simulink model "VTOL_quadplane"  (R2026a)
settings: Solver=ode1  StopTime=120  FixedStep=1/60  MaxStep=0.01
undefined symbols (not defined in the file or in its folder): op_trim, params, Receive, Send
libraries: slpidlib x32, simulink_extras x11, simulink x2, aerolibfltsims x2, aerolibobsolete x1, sim3dlib x1, uavsim3dlib x1
(part 2 of 4)

== system VTOL_quadplane/Gravity_forces ==
  DCM : Inport
  Constant2 : Constant  Value=[0;0;params.geometric.mass*params.constants.g]
  MatrixMultiply : Product  Multiplication=Matrix(*)
  Gravity_forces : Outport
  wires:
  DCM/1 -> MatrixMultiply/1
  Constant2/1 -> MatrixMultiply/2
  MatrixMultiply/1 -> Gravity_forces/1

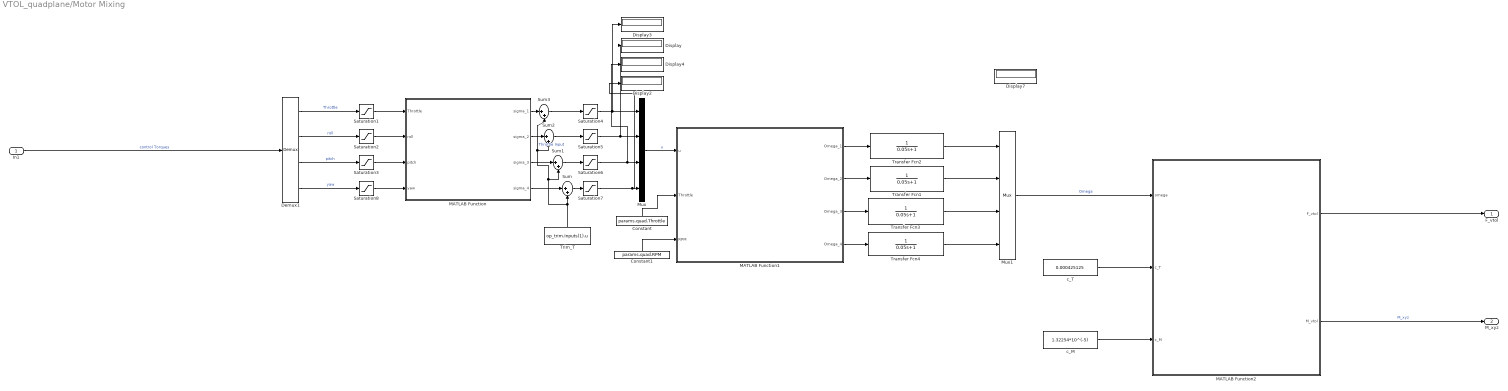
== system VTOL_quadplane/Motor Mixing ==
  In1 : Inport
  Constant : Constant  Value=params.quad.Throttle
  Constant1 : Constant  Value=params.quad.RPM
  Demux1 : Demux
  Display{,2..4,7} (5 alike) : Display
  MATLAB Function : MATLAB Function  TreatAsAtomicUnit=on
  MATLAB Function1 : MATLAB Function  TreatAsAtomicUnit=on
  MATLAB Function2 : MATLAB Function  TreatAsAtomicUnit=on
  Mux : Mux
  Mux1 : Mux
  Saturation1 : Saturate  UpperLimit=0.15  LowerLimit=-0.15
  Saturation2 : Saturate  UpperLimit=0.15  LowerLimit=-0.15
  Saturation3 : Saturate  UpperLimit=0.15  LowerLimit=-0.15
  Saturation{4..7} (4 alike) : Saturate  UpperLimit=0.9  LowerLimit=0.1
  Saturation8 : Saturate  UpperLimit=0.05  LowerLimit=-0.05
  Sum{,1..3} (4 alike) : Sum  Inputs=|++
  Transfer Fcn{1..4} (4 alike) : TransferFcn  Denominator=[0.05 1]
  Trim_T : Constant  Value=op_trim.Inputs(1).u
  c_M : Constant  Value=1.32254*10^(-5)
  c_T : Constant  Value=0.000425125
  F_vtol : Outport
  M_xyz : Outport  Port=2
  wires:
  Saturation4/1 -> Display3/1, Mux/1
  Demux1/4 -> Saturation8/1  "yaw"
  Constant/1 -> MATLAB Function1/2(Throttle)
  MATLAB Function1/3(Omega_3) -> Transfer Fcn3/1
  MATLAB Function1/1(Omega_1) -> Transfer Fcn2/1
  MATLAB Function1/2(Omega_2) -> Transfer Fcn1/1
  MATLAB Function1/4(Omega_4) -> Transfer Fcn4/1
  Mux1/1 -> MATLAB Function2/1(omega)  "Omega"
  Saturation7/1 -> Display2/1, Mux/4
  Demux1/1 -> Saturation1/1  "Throttle"
  Demux1/3 -> Saturation3/1  "pitch"
  MATLAB Function2/2(M_vtol) -> M_xyz/1  "M_xyz"
  Mux/1 -> MATLAB Function1/1(u)  "u"
  Demux1/2 -> Saturation2/1  "roll"
  In1/1 -> Demux1/1  "control Torques"
  Saturation5/1 -> Display/1, Mux/2
  Constant1/1 -> MATLAB Function1/3(RPM)
  Saturation6/1 -> Display4/1, Mux/3
  c_M/1 -> MATLAB Function2/3(c_M)
  c_T/1 -> MATLAB Function2/2(c_T)
  MATLAB Function2/1(F_vtol) -> F_vtol/1
  Transfer Fcn2/1 -> Mux1/1
  Transfer Fcn1/1 -> Mux1/2
  Transfer Fcn3/1 -> Mux1/3
  Transfer Fcn4/1 -> Mux1/4
  Sum/1 -> Saturation7/1
  Trim_T/1 -> Sum1/2, Sum3/2, Sum2/2, Sum/2  "Throttle Input"
  MATLAB Function/1(sigma_1) -> Sum3/1
  MATLAB Function/2(sigma_2) -> Sum2/1
  MATLAB Function/3(sigma_3) -> Sum1/1
  MATLAB Function/4(sigma_4) -> Sum/1
  Sum1/1 -> Saturation6/1
  Sum2/1 -> Saturation5/1
  Sum3/1 -> Saturation4/1
  Saturation1/1 -> MATLAB Function/1(Throttle)
  Saturation2/1 -> MATLAB Function/2(roll)
  Saturation3/1 -> MATLAB Function/3(pitch)
  Saturation8/1 -> MATLAB Function/4(yaw)

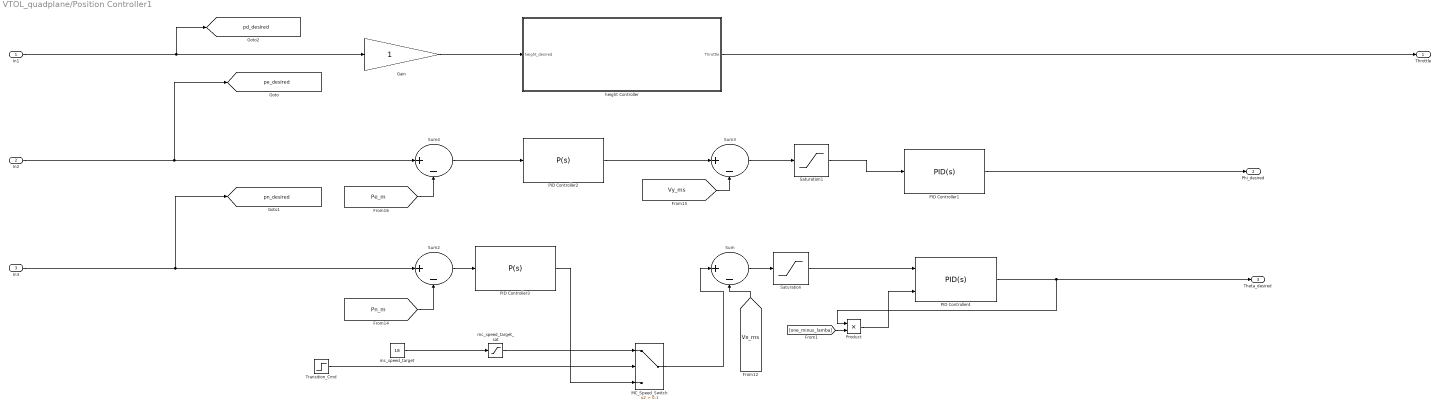
== system VTOL_quadplane/Position Controller1 ==
  In1 : Inport
  In2 : Inport  Port=2
  In3 : Inport  Port=3
  Gain : Gain
  MC_Speed_Switch : Switch  Criteria=u2 > Threshold  Threshold=0.1  SaturateOnIntegerOverflow=off  InputSameDT=off
  PID Controller1 : slpidlib/PID Controller  Controller=PID  Form=Parallel  TimeDomain=Continuous-time  UseExternalTs=off  SampleTime=-1  IntegratorMethod=Forward Euler  FilterMethod=Forward Euler  ControllerParametersSource=internal  P=0.103  I=0.0188  UseKiTs=off  D=0.0191  UseExternalDerivativeSource=off  N=100  UseFilter=on  TunerSelectOption=Transfer Function Based (PID Tuner App)  InitialConditionSource=internal  InitialConditionForIntegrator=0  InitialConditionForFilter=0  DifferentiatorICPrevScaledInput=0  ExternalReset=none  TrackingMode=off  Kt=1  LimitOutput=on  SatLimitsSource=internal  UpperSaturationLimit=deg2rad(25)  LowerSaturationLimit=-deg2rad(25)  LinearizeAsGain=on  AntiWindupMode=back-calculation  Kb=1  LimitIntegrator=off  UpperIntegratorSaturationLimit=inf  LowerIntegratorSaturationLimit=-inf  POutMin=[]  POutMax=[]  IOutMin=[]  IOutMax=[]  DOutMin=[]  DOutMax=[]  NOutMin=[]  NOutMax=[]  SumOutMin=[]  SumOutMax=[]  SaturationOutMin=[]  SaturationOutMax=[]  PParamMin=[]  PParamMax=[]  IParamMin=[]  IParamMax=[]  DParamMin=[]  DParamMax=[]  NParamMin=[]  NParamMax=[]  KbParamMin=[]  KbParamMax=[]  KtParamMin=[]  KtParamMax=[]  KbOutMin=[]  KbOutMax=[]  KtOutMin=[]  KtOutMax=[]  IntegratorOutMin=[]  IntegratorOutMax=[]  FilterOutMin=[]  FilterOutMax=[]  SumI1OutMin=[]  SumI1OutMax=[]  SumI2OutMin=[]  SumI2OutMax=[]  SumI3OutMin=[]  SumI3OutMax=[]  SumI4OutMin=[]  SumI4OutMax=[]  SumDOutMin=[]  SumDOutMax=[]  DifferentiatorOutMin=[]  DifferentiatorOutMax=[]  FilterDiffOutCoefMin=[]  FilterDiffOutCoefMax=[]  ReciprocalOutMin=[]  ReciprocalOutMax=[]  SumDenOutMin=[]  SumDenOutMax=[]  SumNumOutMin=[]  SumNumOutMax=[]  DivideOutMin=[]  DivideOutMax=[]  UdiffTsProdOutMin=[]  UdiffTsProdOutMax=[]  NTsProdOutMin=[]  NTsProdOutMax=[]  UintegralTsProdOutMin=[]  UintegralTsProdOutMax=[]  UngainTsProdOutMin=[]  UngainTsProdOutMax=[]  ClampingZeroOutDataTypeStr=Inherit: Inherit via back propagation  ClampingZeroOutMin=[]  ClampingZeroOutMax=[]  FilterDenConstantOutDataTypeStr=Inherit: Inherit via back propagation  FilterDenConstantOutMin=[]  FilterDenConstantOutMax=[]  PCopyOutDataTypeStr=Inherit: Inherit via back propagation  PCopyOutMin=[]  PCopyOutMax=[]  NCopyOutDataTypeStr=Inherit: Inherit via back propagation  NCopyOutMin=[]  NCopyOutMax=[]  IntegratorContinuousStateAttributes=''  IntegratorStateMustResolveToSignalObject=off  IntegratorRTWStateStorageClass=Auto  FilterContinuousStateAttributes=''  FilterStateMustResolveToSignalObject=off  FilterRTWStateStorageClass=Auto  ParallelPVariant=InternalParameters  IdealPVariant=Disabled  IVariant=InternalParameters  DVariant=InternalParameters  IntegratorVariant=Continuous  SatVariant=Enabled  AWVariant=BackCalculation  PCopyVariant=Disabled  TRVariant=Disabled  FdbkBlocksVariant=Forward  IdealPFdbkVariant=Disabled  SatFdbkVariant=Disabled  DerivativeFilterVariant=ContFilter  NVariant=InternalParameters  NCopyVariant=Disabled  FilterICVariant=InternalICsFilter  IntegratorICVariant=InternalICs  ExternalResetVariant=Disabled  TRSumVariant=Passthrough  SumFdbkVariant=Disabled  SumVariant=Sum_PID  TsampFilterVariant=InternalTs  TsampNgainVariant=Passthrough  TsampIntegralVariant=Disabled_SignalSpec  ExternalSaturationOutDataTypeStr=Inherit: Same as second input  DerivativeSourceVariant=ErrorSignal  PreIntVariant=InternalPreInt
  PID Controller2 : slpidlib/PID Controller  Controller=P  Form=Parallel  TimeDomain=Continuous-time  UseExternalTs=off  SampleTime=-1  IntegratorMethod=Forward Euler  FilterMethod=Forward Euler  ControllerParametersSource=internal  P=0.266  I=1  UseKiTs=off  D=0.212  UseExternalDerivativeSource=off  N=100  UseFilter=on  TunerSelectOption=Transfer Function Based (PID Tuner App)  InitialConditionSource=internal  InitialConditionForIntegrator=0  InitialConditionForFilter=0  DifferentiatorICPrevScaledInput=0  ExternalReset=none  TrackingMode=off  Kt=1  LimitOutput=off  SatLimitsSource=internal  UpperSaturationLimit=inf  LowerSaturationLimit=-inf  LinearizeAsGain=on  AntiWindupMode=none  Kb=1  LimitIntegrator=off  UpperIntegratorSaturationLimit=inf  LowerIntegratorSaturationLimit=-inf  POutMin=[]  POutMax=[]  IOutMin=[]  IOutMax=[]  DOutMin=[]  DOutMax=[]  NOutMin=[]  NOutMax=[]  SumOutMin=[]  SumOutMax=[]  SaturationOutMin=[]  SaturationOutMax=[]  PParamMin=[]  PParamMax=[]  IParamMin=[]  IParamMax=[]  DParamMin=[]  DParamMax=[]  NParamMin=[]  NParamMax=[]  KbParamMin=[]  KbParamMax=[]  KtParamMin=[]  KtParamMax=[]  KbOutMin=[]  KbOutMax=[]  KtOutMin=[]  KtOutMax=[]  IntegratorOutMin=[]  IntegratorOutMax=[]  FilterOutMin=[]  FilterOutMax=[]  SumI1OutMin=[]  SumI1OutMax=[]  SumI2OutMin=[]  SumI2OutMax=[]  SumI3OutMin=[]  SumI3OutMax=[]  SumI4OutMin=[]  SumI4OutMax=[]  SumDOutMin=[]  SumDOutMax=[]  DifferentiatorOutMin=[]  DifferentiatorOutMax=[]  FilterDiffOutCoefMin=[]  FilterDiffOutCoefMax=[]  ReciprocalOutMin=[]  ReciprocalOutMax=[]  SumDenOutMin=[]  SumDenOutMax=[]  SumNumOutMin=[]  SumNumOutMax=[]  DivideOutMin=[]  DivideOutMax=[]  UdiffTsProdOutMin=[]  UdiffTsProdOutMax=[]  NTsProdOutMin=[]  NTsProdOutMax=[]  UintegralTsProdOutMin=[]  UintegralTsProdOutMax=[]  UngainTsProdOutMin=[]  UngainTsProdOutMax=[]  ClampingZeroOutDataTypeStr=Inherit: Inherit via back propagation  ClampingZeroOutMin=[]  ClampingZeroOutMax=[]  FilterDenConstantOutDataTypeStr=Inherit: Inherit via back propagation  FilterDenConstantOutMin=[]  FilterDenConstantOutMax=[]  PCopyOutDataTypeStr=Inherit: Inherit via back propagation  PCopyOutMin=[]  PCopyOutMax=[]  NCopyOutDataTypeStr=Inherit: Inherit via back propagation  NCopyOutMin=[]  NCopyOutMax=[]  IntegratorContinuousStateAttributes=''  IntegratorStateMustResolveToSignalObject=off  IntegratorRTWStateStorageClass=Auto  FilterContinuousStateAttributes=''  FilterStateMustResolveToSignalObject=off  FilterRTWStateStorageClass=Auto  ParallelPVariant=InternalParameters  IdealPVariant=Disabled  IVariant=Disabled  DVariant=Disabled  IntegratorVariant=Disabled  SatVariant=Disabled  AWVariant=Disabled  PCopyVariant=Disabled  TRVariant=Disabled  FdbkBlocksVariant=Forward  IdealPFdbkVariant=Disabled  SatFdbkVariant=Disabled  DerivativeFilterVariant=Disabled  NVariant=Disabled  NCopyVariant=Disabled_SignalSpec  FilterICVariant=Disabled  IntegratorICVariant=Disabled  ExternalResetVariant=Disabled  TRSumVariant=Passthrough  SumFdbkVariant=Disabled  SumVariant=Passthrough_P  TsampFilterVariant=InternalTs  TsampNgainVariant=Passthrough  TsampIntegralVariant=Disabled_SignalSpec  ExternalSaturationOutDataTypeStr=Inherit: Same as second input  DerivativeSourceVariant=Disabled  PreIntVariant=InternalPreInt
  PID Controller3 : slpidlib/PID Controller  Controller=P  Form=Parallel  TimeDomain=Continuous-time  UseExternalTs=off  SampleTime=-1  IntegratorMethod=Forward Euler  FilterMethod=Forward Euler  ControllerParametersSource=internal  P=0.266  I=1  UseKiTs=off  D=0.1  UseExternalDerivativeSource=off  N=100  UseFilter=on  TunerSelectOption=Transfer Function Based (PID Tuner App)  InitialConditionSource=internal  InitialConditionForIntegrator=0  InitialConditionForFilter=0  DifferentiatorICPrevScaledInput=0  ExternalReset=none  TrackingMode=off  Kt=1  LimitOutput=off  SatLimitsSource=internal  UpperSaturationLimit=inf  LowerSaturationLimit=-inf  LinearizeAsGain=on  AntiWindupMode=none  Kb=1  LimitIntegrator=off  UpperIntegratorSaturationLimit=inf  LowerIntegratorSaturationLimit=-inf  POutMin=[]  POutMax=[]  IOutMin=[]  IOutMax=[]  DOutMin=[]  DOutMax=[]  NOutMin=[]  NOutMax=[]  SumOutMin=[]  SumOutMax=[]  SaturationOutMin=[]  SaturationOutMax=[]  PParamMin=[]  PParamMax=[]  IParamMin=[]  IParamMax=[]  DParamMin=[]  DParamMax=[]  NParamMin=[]  NParamMax=[]  KbParamMin=[]  KbParamMax=[]  KtParamMin=[]  KtParamMax=[]  KbOutMin=[]  KbOutMax=[]  KtOutMin=[]  KtOutMax=[]  IntegratorOutMin=[]  IntegratorOutMax=[]  FilterOutMin=[]  FilterOutMax=[]  SumI1OutMin=[]  SumI1OutMax=[]  SumI2OutMin=[]  SumI2OutMax=[]  SumI3OutMin=[]  SumI3OutMax=[]  SumI4OutMin=[]  SumI4OutMax=[]  SumDOutMin=[]  SumDOutMax=[]  DifferentiatorOutMin=[]  DifferentiatorOutMax=[]  FilterDiffOutCoefMin=[]  FilterDiffOutCoefMax=[]  ReciprocalOutMin=[]  ReciprocalOutMax=[]  SumDenOutMin=[]  SumDenOutMax=[]  SumNumOutMin=[]  SumNumOutMax=[]  DivideOutMin=[]  DivideOutMax=[]  UdiffTsProdOutMin=[]  UdiffTsProdOutMax=[]  NTsProdOutMin=[]  NTsProdOutMax=[]  UintegralTsProdOutMin=[]  UintegralTsProdOutMax=[]  UngainTsProdOutMin=[]  UngainTsProdOutMax=[]  ClampingZeroOutDataTypeStr=Inherit: Inherit via back propagation  ClampingZeroOutMin=[]  ClampingZeroOutMax=[]  FilterDenConstantOutDataTypeStr=Inherit: Inherit via back propagation  FilterDenConstantOutMin=[]  FilterDenConstantOutMax=[]  PCopyOutDataTypeStr=Inherit: Inherit via back propagation  PCopyOutMin=[]  PCopyOutMax=[]  NCopyOutDataTypeStr=Inherit: Inherit via back propagation  NCopyOutMin=[]  NCopyOutMax=[]  IntegratorContinuousStateAttributes=''  IntegratorStateMustResolveToSignalObject=off  IntegratorRTWStateStorageClass=Auto  FilterContinuousStateAttributes=''  FilterStateMustResolveToSignalObject=off  FilterRTWStateStorageClass=Auto  ParallelPVariant=InternalParameters  IdealPVariant=Disabled  IVariant=Disabled  DVariant=Disabled  IntegratorVariant=Disabled  SatVariant=Disabled  AWVariant=Disabled  PCopyVariant=Disabled  TRVariant=Disabled  FdbkBlocksVariant=Forward  IdealPFdbkVariant=Disabled  SatFdbkVariant=Disabled  DerivativeFilterVariant=Disabled  NVariant=Disabled  NCopyVariant=Disabled_SignalSpec  FilterICVariant=Disabled  IntegratorICVariant=Disabled  ExternalResetVariant=Disabled  TRSumVariant=Passthrough  SumFdbkVariant=Disabled  SumVariant=Passthrough_P  TsampFilterVariant=InternalTs  TsampNgainVariant=Passthrough  TsampIntegralVariant=Disabled_SignalSpec  ExternalSaturationOutDataTypeStr=Inherit: Same as second input  DerivativeSourceVariant=Disabled  PreIntVariant=InternalPreInt
  PID Controller4 : slpidlib/PID Controller  Controller=PID  Form=Parallel  TimeDomain=Continuous-time  UseExternalTs=off  SampleTime=-1  IntegratorMethod=Forward Euler  FilterMethod=Forward Euler  ControllerParametersSource=internal  P=-0.102  I=-0.0188  UseKiTs=off  D=-0.0191  UseExternalDerivativeSource=off  N=100  UseFilter=on  TunerSelectOption=Transfer Function Based (PID Tuner App)  InitialConditionSource=internal  InitialConditionForIntegrator=0  InitialConditionForFilter=0  DifferentiatorICPrevScaledInput=0  ExternalReset=none  TrackingMode=on  Kt=1  LimitOutput=on  SatLimitsSource=internal  UpperSaturationLimit=deg2rad(25)  LowerSaturationLimit=-deg2rad(25)  LinearizeAsGain=on  AntiWindupMode=back-calculation  Kb=1  LimitIntegrator=off  UpperIntegratorSaturationLimit=inf  LowerIntegratorSaturationLimit=-inf  POutMin=[]  POutMax=[]  IOutMin=[]  IOutMax=[]  DOutMin=[]  DOutMax=[]  NOutMin=[]  NOutMax=[]  SumOutMin=[]  SumOutMax=[]  SaturationOutMin=[]  SaturationOutMax=[]  PParamMin=[]  PParamMax=[]  IParamMin=[]  IParamMax=[]  DParamMin=[]  DParamMax=[]  NParamMin=[]  NParamMax=[]  KbParamMin=[]  KbParamMax=[]  KtParamMin=[]  KtParamMax=[]  KbOutMin=[]  KbOutMax=[]  KtOutMin=[]  KtOutMax=[]  IntegratorOutMin=[]  IntegratorOutMax=[]  FilterOutMin=[]  FilterOutMax=[]  SumI1OutMin=[]  SumI1OutMax=[]  SumI2OutMin=[]  SumI2OutMax=[]  SumI3OutMin=[]  SumI3OutMax=[]  SumI4OutMin=[]  SumI4OutMax=[]  SumDOutMin=[]  SumDOutMax=[]  DifferentiatorOutMin=[]  DifferentiatorOutMax=[]  FilterDiffOutCoefMin=[]  FilterDiffOutCoefMax=[]  ReciprocalOutMin=[]  ReciprocalOutMax=[]  SumDenOutMin=[]  SumDenOutMax=[]  SumNumOutMin=[]  SumNumOutMax=[]  DivideOutMin=[]  DivideOutMax=[]  UdiffTsProdOutMin=[]  UdiffTsProdOutMax=[]  NTsProdOutMin=[]  NTsProdOutMax=[]  UintegralTsProdOutMin=[]  UintegralTsProdOutMax=[]  UngainTsProdOutMin=[]  UngainTsProdOutMax=[]  ClampingZeroOutDataTypeStr=Inherit: Inherit via back propagation  ClampingZeroOutMin=[]  ClampingZeroOutMax=[]  FilterDenConstantOutDataTypeStr=Inherit: Inherit via back propagation  FilterDenConstantOutMin=[]  FilterDenConstantOutMax=[]  PCopyOutDataTypeStr=Inherit: Inherit via back propagation  PCopyOutMin=[]  PCopyOutMax=[]  NCopyOutDataTypeStr=Inherit: Inherit via back propagation  NCopyOutMin=[]  NCopyOutMax=[]  IntegratorContinuousStateAttributes=''  IntegratorStateMustResolveToSignalObject=off  IntegratorRTWStateStorageClass=Auto  FilterContinuousStateAttributes=''  FilterStateMustResolveToSignalObject=off  FilterRTWStateStorageClass=Auto  ParallelPVariant=InternalParameters  IdealPVariant=Disabled  IVariant=InternalParameters  DVariant=InternalParameters  IntegratorVariant=Continuous  SatVariant=Enabled  AWVariant=BackCalculation  PCopyVariant=Disabled  TRVariant=Enabled  FdbkBlocksVariant=Forward  IdealPFdbkVariant=Disabled  SatFdbkVariant=Disabled  DerivativeFilterVariant=ContFilter  NVariant=InternalParameters  NCopyVariant=Disabled  FilterICVariant=InternalICsFilter  IntegratorICVariant=InternalICs  ExternalResetVariant=Disabled  TRSumVariant=TrackingMode  SumFdbkVariant=Disabled  SumVariant=Sum_PID  TsampFilterVariant=InternalTs  TsampNgainVariant=Passthrough  TsampIntegralVariant=Disabled_SignalSpec  ExternalSaturationOutDataTypeStr=Inherit: Same as second input  DerivativeSourceVariant=ErrorSignal  PreIntVariant=InternalPreInt
  Product : Product
  Saturation : Saturate  UpperLimit=20  LowerLimit=0
  Saturation1 : Saturate  UpperLimit=5  LowerLimit=-5
  Sum{,2..4} (4 alike) : Sum  Inputs=|+-
  Transition_Cmd : Step  Time=10
  height Controller : Subsystem
  mc_speed_target : Constant  Value=18
  mc_speed_target_sat : Saturate  UpperLimit=20  LowerLimit=0
  Throttle : Outport
  Phi_desired : Outport  Port=2
  Theta_desired : Outport  Port=3
  tag scope: pd_desired=global, pe_desired=global, pn_desired=global
  wires:
  Product/1 -> PID Controller4/2
  [one_minus_lamba] -> Product/2
  PID Controller3/1 -> MC_Speed_Switch/3
  mc_speed_target_sat/1 -> MC_Speed_Switch/1
  MC_Speed_Switch/1 -> Sum/1
  mc_speed_target/1 -> mc_speed_target_sat/1
  Transition_Cmd/1 -> MC_Speed_Switch/2
  PID Controller4/1 -> Theta_desired/1, Product/1
  PID Controller1/1 -> Phi_desired/1
  height Controller/1(Throttle) -> Throttle/1
  Saturation/1 -> PID Controller4/1
  Sum4/1 -> PID Controller2/1
  [Pe_m] -> Sum4/2
  Sum2/1 -> PID Controller3/1
  PID Controller2/1 -> Sum3/1
  [Vy_ms] -> Sum3/2
  [Pn_m] -> Sum2/2
  Sum/1 -> Saturation/1
  Sum3/1 -> Saturation1/1
  Saturation1/1 -> PID Controller1/1
  In3/1 -> Sum2/1, [pn_desired]
  [Vx_ms] -> Sum/2
  In2/1 -> Sum4/1, [pe_desired]
  Gain/1 -> height Controller/1(height_desired)
  In1/1 -> Gain/1, [pd_desired]

== system VTOL_quadplane/Quad Velocity Controller ==
  In1 : Inport
  In2 : Inport  Port=2
  In3 : Inport  Port=3
  Gain : Gain
  PID Controller1 : slpidlib/PID Controller  Controller=PID  Form=Parallel  TimeDomain=Continuous-time  UseExternalTs=off  SampleTime=-1  IntegratorMethod=Forward Euler  FilterMethod=Forward Euler  ControllerParametersSource=internal  P=0.103  I=0.0188  UseKiTs=off  D=0.0191  UseExternalDerivativeSource=off  N=100  UseFilter=on  TunerSelectOption=Transfer Function Based (PID Tuner App)  InitialConditionSource=internal  InitialConditionForIntegrator=0  InitialConditionForFilter=0  DifferentiatorICPrevScaledInput=0  ExternalReset=none  TrackingMode=off  Kt=1  LimitOutput=on  SatLimitsSource=internal  UpperSaturationLimit=deg2rad(25)  LowerSaturationLimit=-deg2rad(25)  LinearizeAsGain=on  AntiWindupMode=back-calculation  Kb=1  LimitIntegrator=off  UpperIntegratorSaturationLimit=inf  LowerIntegratorSaturationLimit=-inf  POutMin=[]  POutMax=[]  IOutMin=[]  IOutMax=[]  DOutMin=[]  DOutMax=[]  NOutMin=[]  NOutMax=[]  SumOutMin=[]  SumOutMax=[]  SaturationOutMin=[]  SaturationOutMax=[]  PParamMin=[]  PParamMax=[]  IParamMin=[]  IParamMax=[]  DParamMin=[]  DParamMax=[]  NParamMin=[]  NParamMax=[]  KbParamMin=[]  KbParamMax=[]  KtParamMin=[]  KtParamMax=[]  KbOutMin=[]  KbOutMax=[]  KtOutMin=[]  KtOutMax=[]  IntegratorOutMin=[]  IntegratorOutMax=[]  FilterOutMin=[]  FilterOutMax=[]  SumI1OutMin=[]  SumI1OutMax=[]  SumI2OutMin=[]  SumI2OutMax=[]  SumI3OutMin=[]  SumI3OutMax=[]  SumI4OutMin=[]  SumI4OutMax=[]  SumDOutMin=[]  SumDOutMax=[]  DifferentiatorOutMin=[]  DifferentiatorOutMax=[]  FilterDiffOutCoefMin=[]  FilterDiffOutCoefMax=[]  ReciprocalOutMin=[]  ReciprocalOutMax=[]  SumDenOutMin=[]  SumDenOutMax=[]  SumNumOutMin=[]  SumNumOutMax=[]  DivideOutMin=[]  DivideOutMax=[]  UdiffTsProdOutMin=[]  UdiffTsProdOutMax=[]  NTsProdOutMin=[]  NTsProdOutMax=[]  UintegralTsProdOutMin=[]  UintegralTsProdOutMax=[]  UngainTsProdOutMin=[]  UngainTsProdOutMax=[]  ClampingZeroOutDataTypeStr=Inherit: Inherit via back propagation  ClampingZeroOutMin=[]  ClampingZeroOutMax=[]  FilterDenConstantOutDataTypeStr=Inherit: Inherit via back propagation  FilterDenConstantOutMin=[]  FilterDenConstantOutMax=[]  PCopyOutDataTypeStr=Inherit: Inherit via back propagation  PCopyOutMin=[]  PCopyOutMax=[]  NCopyOutDataTypeStr=Inherit: Inherit via back propagation  NCopyOutMin=[]  NCopyOutMax=[]  IntegratorContinuousStateAttributes=''  IntegratorStateMustResolveToSignalObject=off  IntegratorRTWStateStorageClass=Auto  FilterContinuousStateAttributes=''  FilterStateMustResolveToSignalObject=off  FilterRTWStateStorageClass=Auto  ParallelPVariant=InternalParameters  IdealPVariant=Disabled  IVariant=InternalParameters  DVariant=InternalParameters  IntegratorVariant=Continuous  SatVariant=Enabled  AWVariant=BackCalculation  PCopyVariant=Disabled  TRVariant=Disabled  FdbkBlocksVariant=Forward  IdealPFdbkVariant=Disabled  SatFdbkVariant=Disabled  DerivativeFilterVariant=ContFilter  NVariant=InternalParameters  NCopyVariant=Disabled  FilterICVariant=InternalICsFilter  IntegratorICVariant=InternalICs  ExternalResetVariant=Disabled  TRSumVariant=Passthrough  SumFdbkVariant=Disabled  SumVariant=Sum_PID  TsampFilterVariant=InternalTs  TsampNgainVariant=Passthrough  TsampIntegralVariant=Disabled_SignalSpec  ExternalSaturationOutDataTypeStr=Inherit: Same as second input  DerivativeSourceVariant=ErrorSignal  PreIntVariant=InternalPreInt
  PID Controller4 : slpidlib/PID Controller  Controller=PID  Form=Parallel  TimeDomain=Continuous-time  UseExternalTs=off  SampleTime=-1  IntegratorMethod=Forward Euler  FilterMethod=Forward Euler  ControllerParametersSource=internal  P=-0.102  I=-0.0188  UseKiTs=off  D=-0.0191  UseExternalDerivativeSource=off  N=100  UseFilter=on  TunerSelectOption=Transfer Function Based (PID Tuner App)  InitialConditionSource=internal  InitialConditionForIntegrator=0  InitialConditionForFilter=0  DifferentiatorICPrevScaledInput=0  ExternalReset=none  TrackingMode=on  Kt=1  LimitOutput=on  SatLimitsSource=internal  UpperSaturationLimit=deg2rad(25)  LowerSaturationLimit=-deg2rad(25)  LinearizeAsGain=on  AntiWindupMode=back-calculation  Kb=1  LimitIntegrator=off  UpperIntegratorSaturationLimit=inf  LowerIntegratorSaturationLimit=-inf  POutMin=[]  POutMax=[]  IOutMin=[]  IOutMax=[]  DOutMin=[]  DOutMax=[]  NOutMin=[]  NOutMax=[]  SumOutMin=[]  SumOutMax=[]  SaturationOutMin=[]  SaturationOutMax=[]  PParamMin=[]  PParamMax=[]  IParamMin=[]  IParamMax=[]  DParamMin=[]  DParamMax=[]  NParamMin=[]  NParamMax=[]  KbParamMin=[]  KbParamMax=[]  KtParamMin=[]  KtParamMax=[]  KbOutMin=[]  KbOutMax=[]  KtOutMin=[]  KtOutMax=[]  IntegratorOutMin=[]  IntegratorOutMax=[]  FilterOutMin=[]  FilterOutMax=[]  SumI1OutMin=[]  SumI1OutMax=[]  SumI2OutMin=[]  SumI2OutMax=[]  SumI3OutMin=[]  SumI3OutMax=[]  SumI4OutMin=[]  SumI4OutMax=[]  SumDOutMin=[]  SumDOutMax=[]  DifferentiatorOutMin=[]  DifferentiatorOutMax=[]  FilterDiffOutCoefMin=[]  FilterDiffOutCoefMax=[]  ReciprocalOutMin=[]  ReciprocalOutMax=[]  SumDenOutMin=[]  SumDenOutMax=[]  SumNumOutMin=[]  SumNumOutMax=[]  DivideOutMin=[]  DivideOutMax=[]  UdiffTsProdOutMin=[]  UdiffTsProdOutMax=[]  NTsProdOutMin=[]  NTsProdOutMax=[]  UintegralTsProdOutMin=[]  UintegralTsProdOutMax=[]  UngainTsProdOutMin=[]  UngainTsProdOutMax=[]  ClampingZeroOutDataTypeStr=Inherit: Inherit via back propagation  ClampingZeroOutMin=[]  ClampingZeroOutMax=[]  FilterDenConstantOutDataTypeStr=Inherit: Inherit via back propagation  FilterDenConstantOutMin=[]  FilterDenConstantOutMax=[]  PCopyOutDataTypeStr=Inherit: Inherit via back propagation  PCopyOutMin=[]  PCopyOutMax=[]  NCopyOutDataTypeStr=Inherit: Inherit via back propagation  NCopyOutMin=[]  NCopyOutMax=[]  IntegratorContinuousStateAttributes=''  IntegratorStateMustResolveToSignalObject=off  IntegratorRTWStateStorageClass=Auto  FilterContinuousStateAttributes=''  FilterStateMustResolveToSignalObject=off  FilterRTWStateStorageClass=Auto  ParallelPVariant=InternalParameters  IdealPVariant=Disabled  IVariant=InternalParameters  DVariant=InternalParameters  IntegratorVariant=Continuous  SatVariant=Enabled  AWVariant=BackCalculation  PCopyVariant=Disabled  TRVariant=Enabled  FdbkBlocksVariant=Forward  IdealPFdbkVariant=Disabled  SatFdbkVariant=Disabled  DerivativeFilterVariant=ContFilter  NVariant=InternalParameters  NCopyVariant=Disabled  FilterICVariant=InternalICsFilter  IntegratorICVariant=InternalICs  ExternalResetVariant=Disabled  TRSumVariant=TrackingMode  SumFdbkVariant=Disabled  SumVariant=Sum_PID  TsampFilterVariant=InternalTs  TsampNgainVariant=Passthrough  TsampIntegralVariant=Disabled_SignalSpec  ExternalSaturationOutDataTypeStr=Inherit: Same as second input  DerivativeSourceVariant=ErrorSignal  PreIntVariant=InternalPreInt
  Product : Product
  Saturation : Saturate  UpperLimit=25  LowerLimit=-25
  Saturation1 : Saturate  UpperLimit=20  LowerLimit=-20
  Sum : Sum  Inputs=|+-
  Sum3 : Sum  Inputs=|+-
  height Controller : Subsystem
  Throttle : Outport
  Phi_desired : Outport  Port=2
  Theta_desired : Outport  Port=3
  tag scope: pd_desired=global
  wires:
  In1/1 -> [pd_desired], Gain/1
  Gain/1 -> height Controller/1(height_desired)
  Saturation1/1 -> PID Controller1/1
  Sum3/1 -> Saturation1/1
  Sum/1 -> Saturation/1
  [Vy_ms] -> Sum3/2
  In2/1 -> Sum3/1
  Saturation/1 -> PID Controller4/1
  height Controller/1(Throttle) -> Throttle/1
  PID Controller1/1 -> Phi_desired/1
  PID Controller4/1 -> Product/1, Theta_desired/1
  [one_minus_lambda] -> Product/2
  Product/1 -> ?
  In3/1 -> Sum/1
  [Vx_ms] -> Sum/2

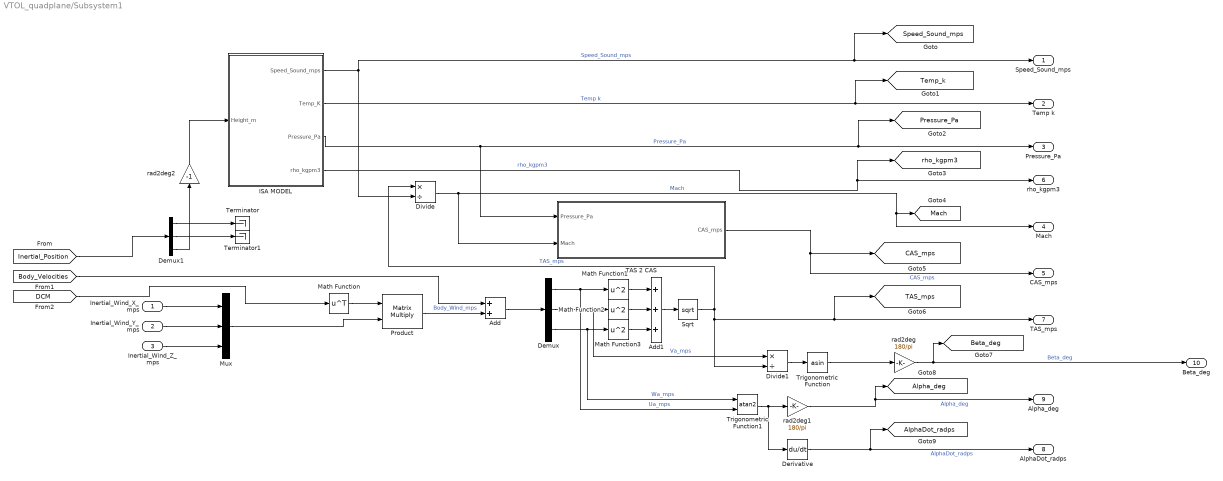
== system VTOL_quadplane/Subsystem1 ==
  Inertial_Wind_X_mps : Inport
  Inertial_Wind_Y_mps : Inport  Port=2
  Inertial_Wind_Z_mps : Inport  Port=3
  Add : Sum
  Add1 : Sum  Inputs=+++
  Demux : Demux  Outputs=3
  Demux1 : Demux  Outputs=3
  Derivative : Derivative
  Divide : Product  Inputs=*/
  Divide1 : Product  Inputs=*/
  ISA MODEL : Subsystem
  Math Function : Math  Operator=transpose  SignedPower=on
  Math Function1 : Math  Operator=square  SignedPower=on
  Math Function2 : Math  Operator=square  SignedPower=on
  Math Function3 : Math  Operator=square  SignedPower=on
  Mux : Mux  Inputs=3
  Product : Product  Multiplication=Matrix(*)
  Sqrt : Sqrt
  TAS 2 CAS : Subsystem
  Terminator : Terminator
  Terminator1 : Terminator
  Trigonometric Function : Trigonometry  Operator=asin
  Trigonometric Function1 : Trigonometry  Operator=atan2
  rad2deg : Gain  Gain=180/pi
  rad2deg1 : Gain  Gain=180/pi
  rad2deg2 : Gain  Gain=-1
  Speed_Sound_mps : Outport
  Temp k : Outport  Port=2
  Pressure_Pa : Outport  Port=3
  Mach : Outport  Port=4
  CAS_mps : Outport  Port=5
  rho_kgpm3 : Outport  Port=6
  TAS_mps : Outport  Port=7
  AlphaDot_radps : Outport  Port=8
  Alpha_deg : Outport  Port=9
  Beta_deg : Outport  Port=10
  tag scope: AlphaDot_radps=global, Alpha_deg=global, Beta_deg=global, CAS_mps=global, Mach=global, Pressure_Pa=global, Speed_Sound_mps=global, TAS_mps=global, Temp_k=global, rho_kgpm3=global
  wires:
  Sqrt/1 -> Divide/1, [TAS_mps], TAS_mps/1, Divide1/2  "TAS_mps"
  [Inertial_Position] -> Demux1/1
  ISA MODEL/2(Temp_K) -> Temp k/1, [Temp_k]  "Temp k"
  Demux1/3 -> rad2deg2/1
  [Body_Velocities] -> Add/1
  ISA MODEL/3(Pressure_Pa) -> TAS 2 CAS/1(Pressure_Pa), [Pressure_Pa], Pressure_Pa/1  "Pressure_Pa"
  TAS 2 CAS/1(CAS_mps) -> CAS_mps/1, [CAS_mps]  "CAS_mps"
  rad2deg2/1 -> ISA MODEL/1("Height_m ")
  Math Function1/1 -> Add1/1
  Divide/1 -> TAS 2 CAS/2(Mach), Mach/1, [Mach]  "Mach"
  ISA MODEL/1(Speed_Sound_mps) -> Speed_Sound_mps/1, [Speed_Sound_mps], Divide/2  "Speed_Sound_mps"
  Inertial_Wind_Y_mps/1 -> Mux/2
  Demux/3 -> Math Function3/1, Trigonometric Function1/1  "Wa_mps"
  Demux/1 -> Math Function1/1, Trigonometric Function1/2  "Ua_mps"
  Derivative/1 -> AlphaDot_radps/1, [AlphaDot_radps]  "AlphaDot_radps"
  Math Function3/1 -> Add1/3
  Demux1/2 -> Terminator1/1
  Product/1 -> Add/2  "Body_Wind_mps"
  Demux/2 -> Math Function2/1, Divide1/1  "Va_mps"
  [DCM] -> Math Function/1
  Divide1/1 -> Trigonometric Function/1
  Add1/1 -> Sqrt/1
  Trigonometric Function1/1 -> rad2deg1/1, Derivative/1
  Mux/1 -> Product/2
  Demux1/1 -> Terminator/1
  ISA MODEL/4(rho_kgpm3) -> [rho_kgpm3], rho_kgpm3/1  "rho_kgpm3"
  Inertial_Wind_Z_mps/1 -> Mux/3
  rad2deg/1 -> [Beta_deg], Beta_deg/1  "Beta_deg"
  Math Function/1 -> Product/1
  Trigonometric Function/1 -> rad2deg/1
  Inertial_Wind_X_mps/1 -> Mux/1
  rad2deg1/1 -> Alpha_deg/1, [Alpha_deg]  "Alpha_deg"
  Add/1 -> Demux/1
  Math Function2/1 -> Add1/2

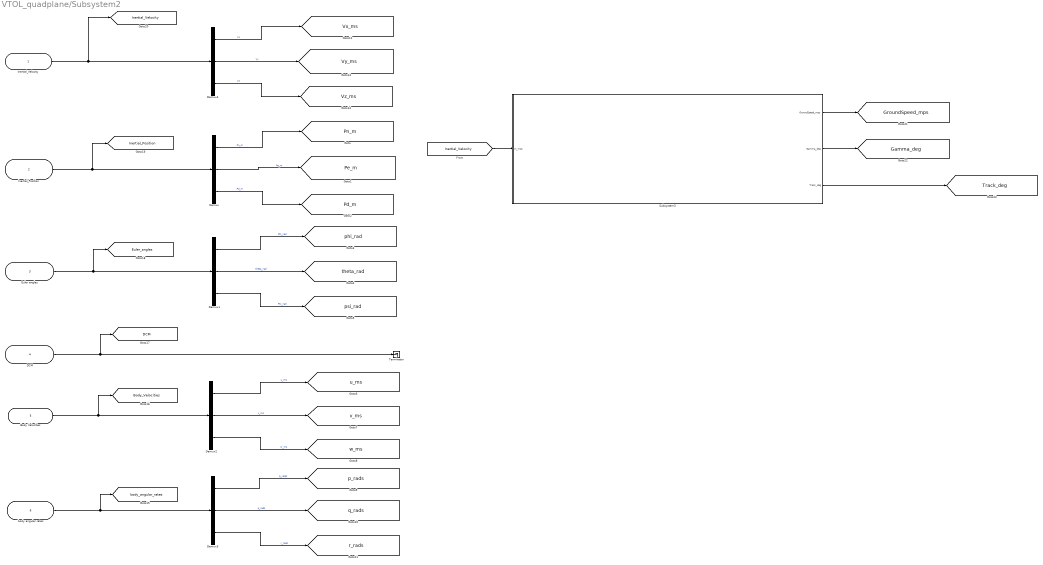
== system VTOL_quadplane/Subsystem2 ==
  Inertial_Velocity : Inport
  Inertial_Position : Inport  Port=2
  Euler angles : Inport  Port=3
  DCM : Inport  Port=4
  Body Velocities : Inport  Port=5
  body angular rates : Inport  Port=6
  Demux{,1..4} (5 alike) : Demux  Outputs=3
  Subsystem3 : Subsystem
  Terminator : Terminator
  tag scope: Body_Velocities=global, DCM=global, Euler_angles=global, Gamma_deg=global, GroundSpeed_mps=global, Inertial_Position=global, Inertial_Velocity=global, Pd_m=global, Pe_m=global, Pn_m=global, Track_deg=global, Vx_ms=global, Vy_ms=global, Vz_ms=global, body_angular_rates=global, p_rads=global, phi_rad=global, psi_rad=global, q_rads=global, r_rads=global, theta_rad=global, u_ms=global, v_ms=global, w_ms=global
  wires:
  Demux3/3 -> [r_rads]  "r_rads"
  Euler angles/1 -> [Euler_angles], Demux1/1
  Demux2/3 -> [w_ms]  "w_ms"
  Demux2/1 -> [u_ms]  "u_ms"
  Demux1/2 -> [theta_rad]  "theta_rad"
  Demux3/2 -> [q_rads]  "q_rads"
  Inertial_Position/1 -> [Inertial_Position], Demux/1
  Demux2/2 -> [v_ms]  "v_ms"
  Demux1/3 -> [psi_rad]  "Psi_rad"
  Demux/3 -> [Pd_m]  "Pd_m"
  Demux/2 -> [Pe_m]  "Pe_m"
  body angular rates/1 -> [body_angular_rates], Demux3/1
  Body Velocities/1 -> [Body_Velocities], Demux2/1
  Demux/1 -> [Pn_m]  "Pn_m"
  Demux1/1 -> [phi_rad]  "Phi_rad"
  Demux3/1 -> [p_rads]  "p_rad/s"
  Demux4/2 -> [Vy_ms]  "Vy"
  Demux4/3 -> [Vz_ms]  "Vz"
  Demux4/1 -> [Vx_ms]  "Vx"
  Inertial_Velocity/1 -> [Inertial_Velocity], Demux4/1
  DCM/1 -> [DCM], Terminator/1
  [Inertial_Velocity] -> Subsystem3/1(VI_mps)
  Subsystem3/1(GroundSpeed_mps) -> [GroundSpeed_mps]
  Subsystem3/2(Gamma_deg) -> [Gamma_deg]
  Subsystem3/3(Track_deg) -> [Track_deg]

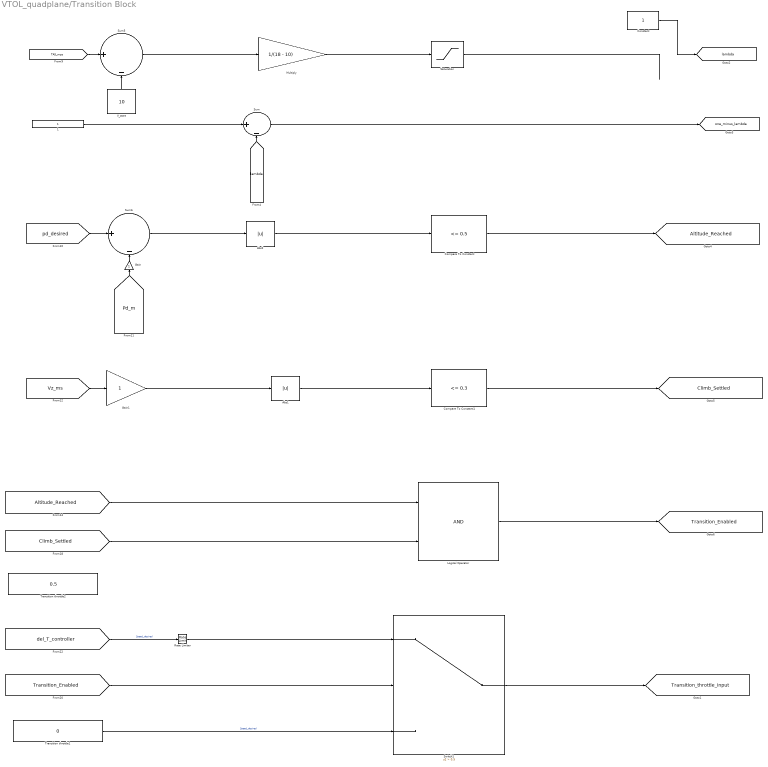
== system VTOL_quadplane/Transition Block ==
  1 : Constant
  Abs1 : Abs  SaturateOnIntegerOverflow=off
  Abs2 : Abs  SaturateOnIntegerOverflow=off
  Compare To Constant : simulink/Logic and Bit Operations/Compare To Constant  relop=<=  const=0.5  OutDataTypeStr=boolean
  Compare To Constant1 : simulink/Logic and Bit Operations/Compare To Constant  relop=<=  const=0.3  OutDataTypeStr=boolean
  Constant : Constant
  Gain : Gain
  Gain1 : Gain
  Logical Operator : Logic  AllPortsSameDT=off  OutDataTypeStr=boolean
  Multiply : Gain  Gain=1/(18 - 10)
  Rate Limiter : RateLimiter  SampleTimeMode=inherited
  Saturation : Saturate  UpperLimit=1  LowerLimit=0
  Sum : Sum  Inputs=|+-
  Sum5 : Sum  Inputs=|+-
  Sum6 : Sum  Inputs=|+-
  Switch1 : Switch  Criteria=u2 > Threshold  Threshold=0.5  SaturateOnIntegerOverflow=off  InputSameDT=off
  Transition throttle1 : Constant  Value=0
  Transition throttle2 : Constant  Value=0.5
  V_start : Constant  Value=10
  tag scope: Altitude_Reached=global, Climb_Settled=global, Transition_Enabled=global, Transition_throttle_input=global, lambda=global, one_minus_lambda=global
  wires:
  Gain/1 -> Sum6/2
  [pd_desired] -> Sum6/1
  Compare To Constant/1 -> [Altitude_Reached]
  [Pd_m] -> Gain/1
  [lambda] -> Sum/2
  Sum5/1 -> Multiply/1
  [TAS_mps] -> Sum5/1
  1/1 -> Sum/1
  V_start/1 -> Sum5/2
  Sum/1 -> [one_minus_lambda]
  Saturation/1 -> ?
  Multiply/1 -> Saturation/1
  Compare To Constant1/1 -> [Climb_Settled]
  Abs1/1 -> Compare To Constant1/1
  Gain1/1 -> Abs1/1
  [Vz_ms] -> Gain1/1
  Switch1/1 -> [Transition_throttle_input]
  [Transition_Enabled] -> Switch1/2
  [Climb_Settled] -> Logical Operator/2
  [Altitude_Reached] -> Logical Operator/1
  Transition throttle1/1 -> Switch1/3  "Speed_desired"
  Rate Limiter/1 -> Switch1/1
  [del_T_controller] -> Rate Limiter/1  "Speed_desired"
  Logical Operator/1 -> [Transition_Enabled]
  Sum6/1 -> Abs2/1
  Abs2/1 -> Compare To Constant/1
  Constant/1 -> [lambda]

== system VTOL_quadplane/Visualisation Subsystem ==
  Translation : Inport
  Rotation : Inport  Port=2
  Constant : Constant  Commented=on
  Demux : Demux  Outputs=3
  Demux1 : Demux  Outputs=3
  Demux2 : Demux  Commented=on  Outputs=2
  Demux3 : Demux  Commented=on  Outputs=3
  Flat Earth to LLA : FlatEarth2LLA  Commented=on
  FlightGear Preconfigured 6DoF Animation : aerolibfltsims/FlightGear Preconfigured 6DoF Animation  Commented=on  xFlightGearVersion=v2019.1  DestinationIpAddress=127.0.0.1  DestinationPort=5502  SampleTime=-1  packetVersion=24
  Gain{,2..4} (4 alike) : Gain  Gain=-1
  Gain1 : Gain
  Gain5 : Gain
  Generate Run Script : aerolibfltsims/Generate Run Script  Commented=on  Architecture=Win64  dataFlow=Send-Receive  GeometryModelName=HL20  AirportId=KSFO  RunwayId=10L  InitialAltitude=7224  InitialHeading=113  OffsetDistance=4.72  OffsetAzimuth=0  InstallScenery=off  DisableShaders=off  OriginAddress=127.0.0.1  DestinationPort=5502  OriginPort=5505  LocalAddress=127.0.0.1  OutputFileName=runfg.bat  FlightGearBaseDirectory=C:\Program Files\FlightGear
  Mux : Mux  Inputs=3
  Mux1 : Mux  Inputs=3
  Mux2 : Mux  Commented=on  Inputs=6
  Simulation 3D Scene Configuration : sim3dlib/Simulation 3D Scene Configuration  Priority=0  ProjectFormat=Default Scenes  SceneDesc=US city block  ProjectName=C:\Program Files\MATLAB\R2026a\toolbox\shared\sim3d_projects\automotive_project_windows\UE\WindowsNoEditor\VehicleSimulation.exe  ScenePath=/Game/Maps/USCityBlock  EnableOpenDRIVE=off  vehTagList={'Custom';'Scene Origin';'SimulinkVehicle1'}  vehTag=SimulinkVehicle1  AttachedCameraRelativeTranslation=[0 0 0]  FreeCameraDefaultInitialTranslation=[-6, 0, 2]  AttachedCameraRelativeRotation=[0, -15, 0]  FreeCameraDefaultInitialRotation=[0, -15, 0]  ViewpointName=Custom  FreeCameraInitialTranslation=[0 0 0]  FreeCameraInitialRotation=[0 0 0]  OpVisEn=off  Ts=1/60  EnableWindow=on  EnableRemoteAccess=off  SimulationMode=CoSimulation  SimulateUsing=Interpreted execution  EnableAnimationRecording=off  OverrideDefaultRecording=off  AnimationRecordingFileName=sim3dAnimation.mat  AnimationRecordingInterval=[0 inf]  EnableWeather=off  SunAzimuth=90  SunAltitude=40.0  EnableGeospatialSun=off  Latitude=0  Longitude=0  Date=2023-01-01  Time=10:30:00  GeoTimeZone=-5.0  SunDaylightSaving=off  wind=1  clouds=10  EnableVolumetricClouds=off  CloudCoverage=0  CloudAltitude=6  fog=0  rain=0  RaindropsEffect=off  SnowDensity=0  EnableGeospatial=off  TilesetSource=Earth terrain  UseTrueOrigin=off  OriginHeight=200  OriginLatitude=40.744652  OriginLongitude=-73.988864  MapStyle=Aerial  AdditionalAssetIDs=[]  UseAdvancedSunSky=off  SolarTime=11  TimeZone=-5  Day=21  Month=9  Year=2022  UseDaylightSavingTime=on  DSTStartDay=10  DSTStartMonth=3  DSTEndDay=3  DSTEndMonth=11  DSTSwitchHour=2  sensorTag=MainCamera1  sensorId=1  sensorName=MainCamera1  mountLoc=Origin  offsetFlag=off  tmountOffset=[0, 0, 0]  rmountOffset=[0, 0, 0]  HorizontalResolution=1280  VerticalResolution=720  HorizontalFOV=60  mountPoint=[0 0 0]  mountOrientation=[0 0 0]  aMode=4  ID=1  GeoTrigger=Inactive  ViewNameList={'Custom'}  ViewTranslationList={'[0 0 0]'}  ViewRotationList={'[0 0 0]'}
      settings: LibrarySourceBlock=uavsim3dlib/Simulation 3D Scene Configuration
  Simulation 3D UAV Vehicle : uavsim3dlib/Simulation 3D UAV Vehicle  Priority=-1  Mesh=Fixed wing  MeshPath=/MathWorksUAVContent/UAVs/HexaRotorUAV/HexaRotor.HexaRotor  Color=Black  ActorName=SimulinkVehicle1  UseGlobalFrame=off  InitialTranslation=[0 0 0]  InitialRotation=[0 0 0]  InitialTranslationGlobal=[0 0 0]  InitialGeoOrigin=[0 0 0]  InitialRotationGlobal=[0 0 0]  SampleTime=-1  ActorType=SimulinkVehicle  ID=1  aMode=4  ActorTag=SimulinkVehicle1
  Terminator : Terminator  Commented=on
  wires:
  Rotation/1 -> Demux3/1, Demux/1
  Mux/1 -> Simulation 3D UAV Vehicle/2
  Demux/3 -> Gain4/1
  Demux/2 -> Gain/1
  Demux1/3 -> Gain2/1
  Translation/1 -> Flat Earth to LLA/1, Demux1/1
  Demux1/2 -> Gain3/1
  Mux1/1 -> Simulation 3D UAV Vehicle/1
  Gain/1 -> Mux/2
  Gain1/1 -> Mux/3
  Gain2/1 -> Mux2/3, Mux1/3  "Altitude"
  Demux1/1 -> Gain5/1
  Gain3/1 -> Mux1/2
  Gain4/1 -> Mux/1
  Gain5/1 -> Mux1/1
  Constant/1 -> Flat Earth to LLA/2
  Flat Earth to LLA/1 -> Demux2/1
  Mux2/1 -> FlightGear Preconfigured 6DoF Animation/1
  Demux2/1 -> Mux2/2  "Longitude"
  Demux2/2 -> Mux2/1  "Latitude"
  Demux3/1 -> Mux2/4  "Phi"
  Demux3/2 -> Mux2/5  "Theta"
  Demux3/3 -> Mux2/6  "Psi"
  Flat Earth to LLA/2 -> Terminator/1

== system VTOL_quadplane/Aero_Forces_and_Moments/CD_s ==
  Add : Sum  Inputs=++++
  Constant : Constant  Value=params.aero.CD0
  Constant2 : Constant  Value=params.aero.CD_de
  Constant3 : Constant  Value=params.geometric.c
  Constant4 : Constant  Value=params.geometric.c
  Constant5 : Constant  Value=params.aero.CD_dAoA
  Constant6 : Constant  Value=params.aero.CD_q
  Divide : Product  Inputs=*/
  Divide1 : Product  Inputs=*/
  Gain : Gain  Gain=2
  Gain1 : Gain  Gain=2
  Product{1..5} (5 alike) : Product
  TAS_Floor1001 : Saturate  UpperLimit=Inf  LowerLimit=0.5
  TAS_Floor1002 : Saturate  UpperLimit=Inf  LowerLimit=0.5
  CD_b : Outport
  wires:
  Constant/1 -> Add/1
  Product1/1 -> Add/2
  Constant2/1 -> Product1/1
  [Del_e] -> Product1/2
  [AlphaDot_radps] -> Product3/1
  Constant3/1 -> Product3/2
  Product3/1 -> Divide1/1
  Gain/1 -> Divide1/2
  Gain1/1 -> Divide/2
  Constant4/1 -> Product5/2
  Product5/1 -> Divide/1
  [q_rads] -> Product5/1
  Product2/1 -> Add/3
  Divide1/1 -> Product2/1
  Constant5/1 -> Product2/2
  Product4/1 -> Add/4
  Divide/1 -> Product4/2
  Constant6/1 -> Product4/1
  Add/1 -> CD_b/1
  TAS_Floor1001/1 -> Gain/1
  TAS_Floor1002/1 -> Gain1/1
  [TAS_mps] -> TAS_Floor1001/1
  [TAS_mps] -> TAS_Floor1002/1

== system VTOL_quadplane/Aero_Forces_and_Moments/CL_b ==
  Add : Sum  Inputs=+++++
  Constant : Constant  Value=params.aero.CL0
  Constant1 : Constant  Value=params.aero.CL_alpha
  Constant2 : Constant  Value=params.aero.CL_de
  Constant3 : Constant  Value=params.geometric.c
  Constant4 : Constant  Value=params.geometric.c
  Constant5 : Constant  Value=params.aero.CL_dAoA
  Constant6 : Constant  Value=params.aero.CL_q
  Divide : Product  Inputs=*/
  Divide1 : Product  Inputs=*/
  Gain : Gain  Gain=2
  Gain1 : Gain  Gain=2
  Product{,1..5} (6 alike) : Product
  TAS_Floor1003 : Saturate  UpperLimit=Inf  LowerLimit=0.5
  TAS_Floor1004 : Saturate  UpperLimit=Inf  LowerLimit=0.5
  CL_b : Outport
  wires:
  Constant/1 -> Add/1
  Product/1 -> Add/2
  Constant1/1 -> Product/1
  [Alpha_rad] -> Product/2
  Product1/1 -> Add/3
  Constant2/1 -> Product1/1
  [Del_e] -> Product1/2
  [AlphaDot_radps] -> Product3/1
  Constant3/1 -> Product3/2
  Product3/1 -> Divide1/1
  Gain/1 -> Divide1/2
  Gain1/1 -> Divide/2
  Constant4/1 -> Product5/2
  Product5/1 -> Divide/1
  [q_rads] -> Product5/1
  Product2/1 -> Add/4
  Divide1/1 -> Product2/1
  Constant5/1 -> Product2/2
  Product4/1 -> Add/5
  Divide/1 -> Product4/2
  Constant6/1 -> Product4/1
  Add/1 -> CL_b/1
  TAS_Floor1003/1 -> Gain/1
  TAS_Floor1004/1 -> Gain1/1
  [TAS_mps] -> TAS_Floor1003/1
  [TAS_mps] -> TAS_Floor1004/1

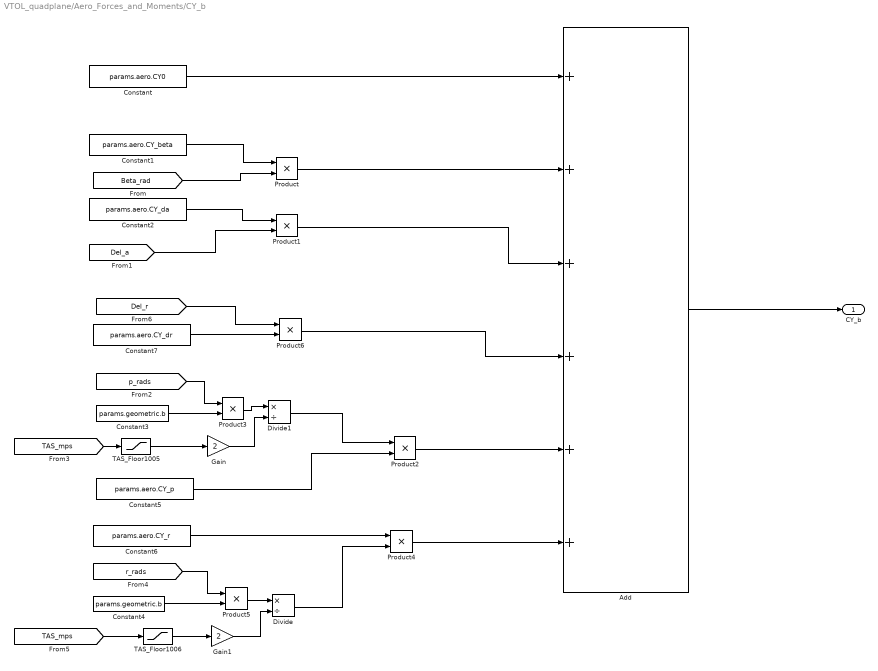
== system VTOL_quadplane/Aero_Forces_and_Moments/CY_b ==
  Add : Sum  Inputs=++++++
  Constant : Constant  Value=params.aero.CY0
  Constant1 : Constant  Value=params.aero.CY_beta
  Constant2 : Constant  Value=params.aero.CY_da
  Constant3 : Constant  Value=params.geometric.b
  Constant4 : Constant  Value=params.geometric.b
  Constant5 : Constant  Value=params.aero.CY_p
  Constant6 : Constant  Value=params.aero.CY_r
  Constant7 : Constant  Value=params.aero.CY_dr
  Divide : Product  Inputs=*/
  Divide1 : Product  Inputs=*/
  Gain : Gain  Gain=2
  Gain1 : Gain  Gain=2
  Product{,1..6} (7 alike) : Product
  TAS_Floor1005 : Saturate  UpperLimit=Inf  LowerLimit=0.5
  TAS_Floor1006 : Saturate  UpperLimit=Inf  LowerLimit=0.5
  CY_b : Outport
  wires:
  Constant/1 -> Add/1
  Product/1 -> Add/2
  Constant1/1 -> Product/1
  [Beta_rad] -> Product/2
  Product1/1 -> Add/3
  Constant2/1 -> Product1/1
  [Del_a] -> Product1/2
  [p_rads] -> Product3/1
  Constant3/1 -> Product3/2
  Product3/1 -> Divide1/1
  Gain/1 -> Divide1/2
  Gain1/1 -> Divide/2
  Constant4/1 -> Product5/2
  Product5/1 -> Divide/1
  [r_rads] -> Product5/1
  Product2/1 -> Add/5
  Divide1/1 -> Product2/1
  Constant5/1 -> Product2/2
  Product4/1 -> Add/6
  Divide/1 -> Product4/2
  Constant6/1 -> Product4/1
  Add/1 -> CY_b/1
  Constant7/1 -> Product6/2
  Product6/1 -> Add/4
  [Del_r] -> Product6/1
  TAS_Floor1005/1 -> Gain/1
  TAS_Floor1006/1 -> Gain1/1
  [TAS_mps] -> TAS_Floor1005/1
  [TAS_mps] -> TAS_Floor1006/1

== system VTOL_quadplane/Aero_Forces_and_Moments/Cl_b ==
  Add : Sum  Inputs=++++++
  Constant : Constant  Value=params.aero.Cl0
  Constant1 : Constant  Value=params.aero.Cl_beta
  Constant2 : Constant  Value=params.aero.Cl_da
  Constant3 : Constant  Value=params.geometric.b
  Constant4 : Constant  Value=params.geometric.b
  Constant5 : Constant  Value=params.aero.Cl_p
  Constant6 : Constant  Value=params.aero.Cl_r
  Constant7 : Constant  Value=params.aero.Cl_dr
  Divide : Product  Inputs=*/
  Divide1 : Product  Inputs=*/
  Gain : Gain  Gain=2
  Gain1 : Gain  Gain=2
  Product{,1..6} (7 alike) : Product
  TAS_Floor1007 : Saturate  UpperLimit=Inf  LowerLimit=0.5
  TAS_Floor1008 : Saturate  UpperLimit=Inf  LowerLimit=0.5
  Cl_b : Outport
  wires:
  [Del_r] -> Product6/1
  Product6/1 -> Add/4
  Constant7/1 -> Product6/2
  Add/1 -> Cl_b/1
  Constant6/1 -> Product4/1
  Divide/1 -> Product4/2
  Product4/1 -> Add/6
  Constant5/1 -> Product2/2
  Divide1/1 -> Product2/1
  Product2/1 -> Add/5
  [r_rads] -> Product5/1
  Product5/1 -> Divide/1
  Constant4/1 -> Product5/2
  Gain1/1 -> Divide/2
  Gain/1 -> Divide1/2
  Product3/1 -> Divide1/1
  Constant3/1 -> Product3/2
  [p_rads] -> Product3/1
  [Del_a] -> Product1/2
  Constant2/1 -> Product1/1
  Product1/1 -> Add/3
  [Beta_rad] -> Product/2
  Constant1/1 -> Product/1
  Product/1 -> Add/2
  Constant/1 -> Add/1
  TAS_Floor1007/1 -> Gain/1
  TAS_Floor1008/1 -> Gain1/1
  [TAS_mps] -> TAS_Floor1008/1
  [TAS_mps] -> TAS_Floor1007/1

== system VTOL_quadplane/Aero_Forces_and_Moments/Cm_b ==
  Add : Sum  Inputs=+++++
  Constant : Constant  Value=params.aero.Cm0
  Constant1 : Constant  Value=params.aero.Cm_alpha
  Constant2 : Constant  Value=params.aero.Cm_de
  Constant3 : Constant  Value=params.geometric.c
  Constant4 : Constant  Value=params.geometric.c
  Constant5 : Constant  Value=params.aero.Cm_dAoA
  Constant6 : Constant  Value=params.aero.Cm_q
  Divide : Product  Inputs=*/
  Divide1 : Product  Inputs=*/
  Gain : Gain  Gain=2
  Gain1 : Gain  Gain=2
  Product{,1..5} (6 alike) : Product
  TAS_Floor1009 : Saturate  UpperLimit=Inf  LowerLimit=0.5
  TAS_Floor1010 : Saturate  UpperLimit=Inf  LowerLimit=0.5
  Cm_b : Outport
  wires:
  Add/1 -> Cm_b/1
  Constant6/1 -> Product4/1
  Divide/1 -> Product4/2
  Product4/1 -> Add/5
  Constant5/1 -> Product2/2
  Divide1/1 -> Product2/1
  Product2/1 -> Add/4
  [q_rads] -> Product5/1
  Product5/1 -> Divide/1
  Constant4/1 -> Product5/2
  Gain1/1 -> Divide/2
  Gain/1 -> Divide1/2
  Product3/1 -> Divide1/1
  Constant3/1 -> Product3/2
  [AlphaDot_radps] -> Product3/1
  [Del_e] -> Product1/2
  Constant2/1 -> Product1/1
  Product1/1 -> Add/3
  [Alpha_rad] -> Product/2
  Constant1/1 -> Product/1
  Product/1 -> Add/2
  Constant/1 -> Add/1
  TAS_Floor1009/1 -> Gain/1
  TAS_Floor1010/1 -> Gain1/1
  [TAS_mps] -> TAS_Floor1009/1
  [TAS_mps] -> TAS_Floor1010/1

== system VTOL_quadplane/Aero_Forces_and_Moments/Cn_b ==
  Add : Sum  Inputs=++++++
  Constant : Constant  Value=params.aero.Cn0
  Constant1 : Constant  Value=params.aero.Cn_beta
  Constant2 : Constant  Value=params.aero.Cn_da
  Constant3 : Constant  Value=params.geometric.b
  Constant4 : Constant  Value=params.geometric.b
  Constant5 : Constant  Value=params.aero.Cn_p
  Constant6 : Constant  Value=params.aero.Cn_r
  Constant7 : Constant  Value=params.aero.Cn_dr
  Divide : Product  Inputs=*/
  Divide1 : Product  Inputs=*/
  Gain : Gain  Gain=2
  Gain1 : Gain  Gain=2
  Product{,1..6} (7 alike) : Product
  TAS_Floor1011 : Saturate  UpperLimit=Inf  LowerLimit=0.5
  TAS_Floor1012 : Saturate  UpperLimit=Inf  LowerLimit=0.5
  Cn_b : Outport
  wires:
  Constant/1 -> Add/1
  Product/1 -> Add/2
  Constant1/1 -> Product/1
  [Beta_rad] -> Product/2
  Product1/1 -> Add/3
  Constant2/1 -> Product1/1
  [Del_a] -> Product1/2
  [p_rads] -> Product3/1
  Constant3/1 -> Product3/2
  Product3/1 -> Divide1/1
  Gain/1 -> Divide1/2
  Gain1/1 -> Divide/2
  Constant4/1 -> Product5/2
  Product5/1 -> Divide/1
  [r_rads] -> Product5/1
  Product2/1 -> Add/5
  Divide1/1 -> Product2/1
  Constant5/1 -> Product2/2
  Product4/1 -> Add/6
  Divide/1 -> Product4/2
  Constant6/1 -> Product4/1
  Add/1 -> Cn_b/1
  Constant7/1 -> Product6/2
  Product6/1 -> Add/4
  [Del_r] -> Product6/1
  TAS_Floor1011/1 -> Gain/1
  TAS_Floor1012/1 -> Gain1/1
  [TAS_mps] -> TAS_Floor1012/1
  [TAS_mps] -> TAS_Floor1011/1

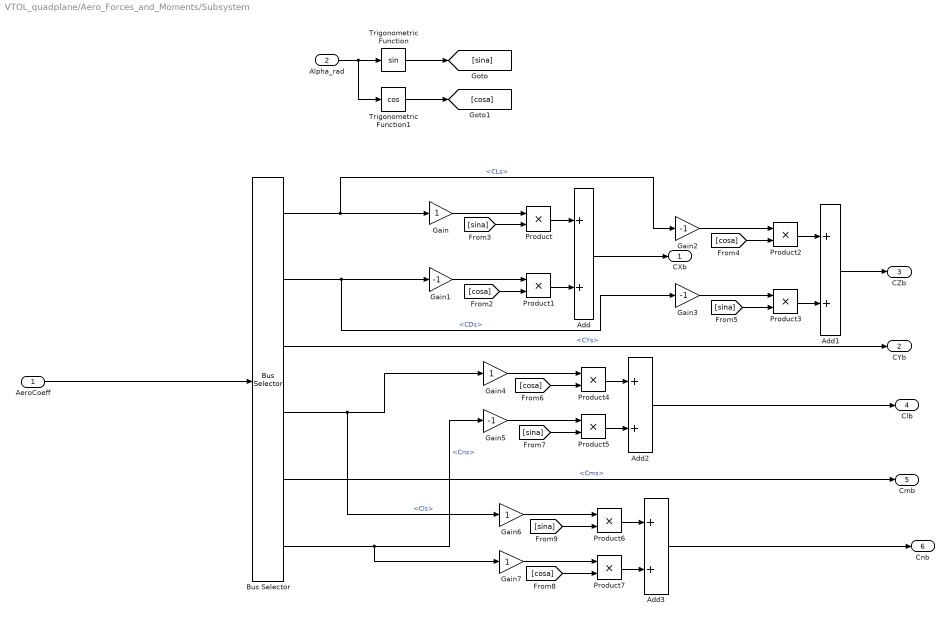
== system VTOL_quadplane/Aero_Forces_and_Moments/Subsystem ==
  AeroCoeff : Inport
  Alpha_rad : Inport  Port=2
  Add{,1..3} (4 alike) : Sum
  Bus Selector : BusSelector  OutputSignals=CLs,CDs,CYs,Cls,Cms,Cns
  Gain{,4,6..7} (4 alike) : Gain
  Gain{1..3,5} (4 alike) : Gain  Gain=-1
  Product{,1..7} (8 alike) : Product
  Trigonometric Function : Trigonometry
  Trigonometric Function1 : Trigonometry  Operator=cos
  CXb : Outport
  CYb : Outport  Port=2
  CZb : Outport  Port=3
  Clb : Outport  Port=4
  Cmb : Outport  Port=5
  Cnb : Outport  Port=6
  wires:
  Product1/1 -> Add/2
  Bus Selector/5 -> Cmb/1  "<Cms>"
  [cosa] -> Product2/2
  Bus Selector/4 -> Gain6/1, Gain4/1  "<Cls>"
  Gain/1 -> Product/1
  Gain1/1 -> Product1/1
  Product3/1 -> Add1/2
  Add2/1 -> Clb/1
  Gain7/1 -> Product7/1
  Bus Selector/3 -> CYb/1  "<CYs>"
  Product2/1 -> Add1/1
  Gain5/1 -> Product5/1
  Product5/1 -> Add2/2
  Gain3/1 -> Product3/1
  Gain2/1 -> Product2/1
  Alpha_rad/1 -> Trigonometric Function1/1, Trigonometric Function/1
  [sina] -> Product6/2
  Product/1 -> Add/1
  Add1/1 -> CZb/1
  Product4/1 -> Add2/1
  Bus Selector/1 -> Gain2/1, Gain/1  "<CLs>"
  Add3/1 -> Cnb/1
  Trigonometric Function/1 -> [sina]
  [sina] -> Product3/2
  AeroCoeff/1 -> Bus Selector/1
  Gain4/1 -> Product4/1
  [cosa] -> Product4/2
  [cosa] -> Product7/2
  Add/1 -> CXb/1
  Bus Selector/2 -> Gain3/1, Gain1/1  "<CDs>"
  Product7/1 -> Add3/2
  Gain6/1 -> Product6/1
  Bus Selector/6 -> Gain7/1, Gain5/1  "<Cns>"
  Trigonometric Function1/1 -> [cosa]
  [cosa] -> Product1/2
  [sina] -> Product/2
  [sina] -> Product5/2
  Product6/1 -> Add3/1

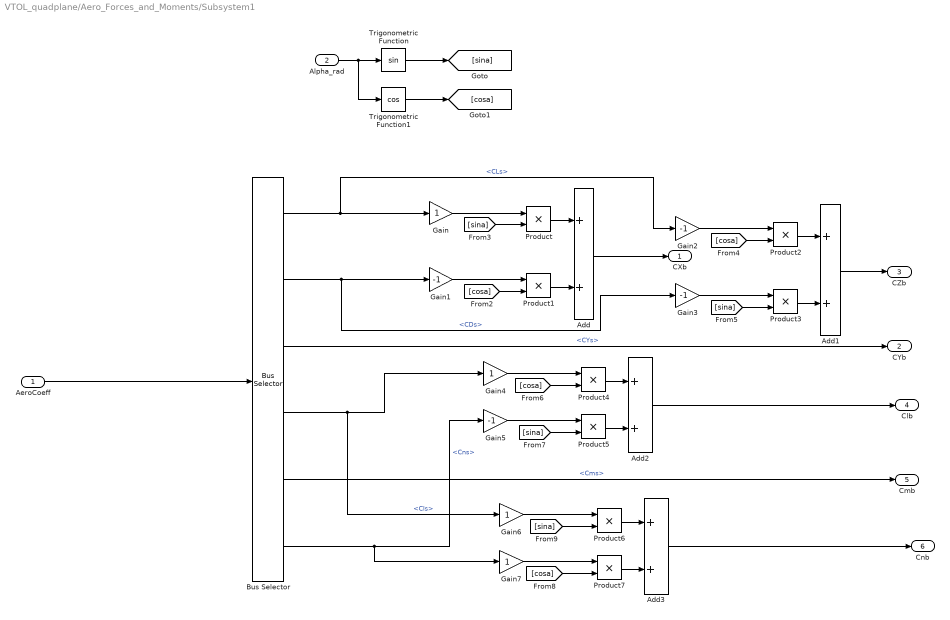
== system VTOL_quadplane/Aero_Forces_and_Moments/Subsystem1 ==
  AeroCoeff : Inport
  Alpha_rad : Inport  Port=2
  Add{,1..3} (4 alike) : Sum
  Bus Selector : BusSelector  OutputSignals=CLs,CDs,CYs,Cls,Cms,Cns
  Gain{,4,6..7} (4 alike) : Gain
  Gain{1..3,5} (4 alike) : Gain  Gain=-1
  Product{,1..7} (8 alike) : Product
  Trigonometric Function : Trigonometry
  Trigonometric Function1 : Trigonometry  Operator=cos
  CXb : Outport
  CYb : Outport  Port=2
  CZb : Outport  Port=3
  Clb : Outport  Port=4
  Cmb : Outport  Port=5
  Cnb : Outport  Port=6
  wires:
  [cosa] -> Product1/2
  Product1/1 -> Add/2
  [sina] -> Product6/2
  [cosa] -> Product4/2
  Bus Selector/4 -> Gain6/1, Gain4/1  "<Cls>"
  Gain/1 -> Product/1
  Bus Selector/3 -> CYb/1  "<CYs>"
  [sina] -> Product/2
  Alpha_rad/1 -> Trigonometric Function1/1, Trigonometric Function/1
  Add3/1 -> Cnb/1
  Product2/1 -> Add1/1
  AeroCoeff/1 -> Bus Selector/1
  Gain3/1 -> Product3/1
  Gain7/1 -> Product7/1
  Product3/1 -> Add1/2
  Product7/1 -> Add3/2
  Gain2/1 -> Product2/1
  Trigonometric Function/1 -> [sina]
  Gain4/1 -> Product4/1
  [sina] -> Product3/2
  Product6/1 -> Add3/1
  Gain1/1 -> Product1/1
  Bus Selector/2 -> Gain3/1, Gain1/1  "<CDs>"
  Bus Selector/6 -> Gain7/1, Gain5/1  "<Cns>"
  Bus Selector/1 -> Gain2/1, Gain/1  "<CLs>"
  [cosa] -> Product7/2
  Product4/1 -> Add2/1
  [sina] -> Product5/2
  Product5/1 -> Add2/2
  Add/1 -> CXb/1
  Add1/1 -> CZb/1
  Product/1 -> Add/1
  Add2/1 -> Clb/1
  [cosa] -> Product2/2
  Gain6/1 -> Product6/1
  Bus Selector/5 -> Cmb/1  "<Cms>"
  Gain5/1 -> Product5/1
  Trigonometric Function1/1 -> [cosa]
